simulink model "AD_Stepper"  (Simulink 10.0)
settings: Solver=FixedStepDiscrete  StartTime=0.0  StopTime=inf  FixedStep=Ts  RelTol=1e-3
PostLoadFcn:
  | Ts = 0.01;      % model sample time
  | Tmax = 0.5;   % maximum time per "tick"
libraries: simulink x4, AD_Stepper_motor_lib x2
settings Model: Creator=Admin  LastModifiedBy=bhisma
settings ConfigSet: Description=rtmc9s12target_R2009b
settings DataIOCC: LimitDataPoints=on  SignalLoggingSaveFormat=ModelDataLogs  SaveOutput=off  SaveTime=off  SignalLoggingName=sigsOut
settings OptimizationCC: ExpressionDepthLimit=2147483647  InitFltsAndDblsToZero=on  LifeSpan=1  EfficientTunableParamExpr=on
settings DebuggingCC: SaveWithParameterizedLinksMsg=none  SignalResolutionControl=TryResolveAllWithWarning  MultiTaskDSMMsg=warning  MultiTaskCondExecSysMsg=none  FcnCallInpInsideContextMsg=warning  StateNameClashWarn=warning
settings HardwareCC: ProdBitPerInt=16  ProdBitPerPointer=16  ProdBitPerSizeT=16  ProdBitPerPtrDiffT=16  ProdEndianess=BigEndian  ProdWordSize=16  ProdHWDeviceType=Motorola HC12
settings SFSimCC: MATLABDynamicMemAlloc=off
settings RTWCC: SystemTargetFile=mc9s12.tlc  GenerateMakefile=off  TemplateMakefile=mc9s12.tmf
settings CodeAppCC: CustomSymbolStrType=$N$R$M  InternalIdentifier=Classic
settings STFCustomTargetCC: TargetFcnLib=ansi_tfl_tmw.mat  ModelReferenceCompliant=off  IncludeMdlTerminateFcn=off  ERTCustomFileBanners=on  SupportNonInlinedSFcns=off  RemoveResetFunc=on  MATLABClassNameForMDSCustomization=Simulink.SoftwareTarget.ERTCustomization  CPPClassGenCompliant=on  SystemTargetFile=mc9s12.tlc
settings ERTTargetCC: TargetFcnLib=ansi_tfl_tmw.mat  MultiwordLength=2048  ModelReferenceCompliant=off  ParMdlRefBuildCompliant=off  CompOptLevelCompliant=off  ConcurrentExecutionCompliant=off  IncludeMdlTerminateFcn=off  CombineOutputUpdateFcns=off  SupportContinuousTime=on  ModelStepFunctionPrototypeControlCompliant=off  GRTInterface=on  UseToolchainInfoCompliant=off  ExtModeMexFile=ext_serial_mc9s12_comm  ExtModeMexArgs=1,2,115200  ERTCustomFileTemplate=mc9s12_file_process.tlc  ConvertIfToSwitch=off  SuppressUnreachableDefaultCases=off
settings CustomProperty: DataType=RTWOptions_EnumType_C__Users_fw__SVN_rtmc9s12-target_trunk_rtmc9s12_CW_R2009b_bin_mc9s12_1mc9s12_TargetBoard  Value=Dragon12Plus
settings EnumStrPairs: String=Dragon12
settings ConfigComp: CovExternalEMLEnable=off

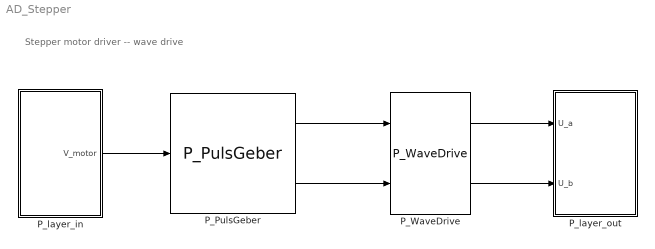
== system AD_Stepper ==
  note: Stepper motor driver -- wave drive
  P_PulsGeber : AD_Stepper_motor_lib/P_PulsGeber  SystemSampleTime=Ts
  P_WaveDrive : AD_Stepper_motor_lib/P_WaveDrive  SystemSampleTime=Ts
  P_layer_in : Subsystem  TreatAsAtomicUnit=on
  P_layer_out : Subsystem  TreatAsAtomicUnit=on  SystemSampleTime=Ts
  wires:
  P_PulsGeber/1 -> P_WaveDrive/1
  P_PulsGeber/2 -> P_WaveDrive/2
  P_layer_in/1(V_motor) -> P_PulsGeber/1
  P_WaveDrive/1 -> P_layer_out/1(U_a)
  P_WaveDrive/2 -> P_layer_out/2(U_b)

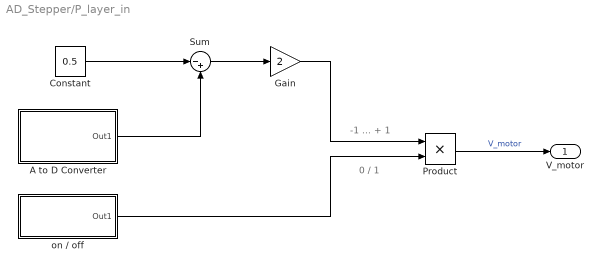
== system AD_Stepper/P_layer_in ==
  note: -1 ... + 1
  note: 0 / 1
  A to D Converter : Subsystem  Tag=mcTarget_adc  mask{bank=0, channels=7, use10bits=10 bits, normalize=max. output:  1, sampletime=Ts}
      mask prompts: bank "ADC bank"; channels "Channels ( 0 - 7 )"; use10bits "ADC resolution"; normalize "Normalization"; sampletime "Sample time"
      mask init:
      | [channelsStr, firstChannel, numChannels] = mbc_adcinput(channels);
      mask Help: web('adc_sfcn_9S12.html');
      mask TypeOptions bank: 0 | 1
      mask TypeOptions use10bits: 10 bits | 8 bits
      mask TypeOptions normalize: raw values | max. output:  1 | max. output:  5
      mask Display: disp(['A to D Converter\n' channelsStr])
  Constant : Constant  Value=0.5
  Gain : Gain  Gain=2
  Product : Product  RndMeth=Zero
  Sum : Sum  Inputs=|-+
  on / off : Subsystem  Tag=mcTarget_digIn  mask{port=Port P, pin=0, sampletime=Ts}
      mask prompts: port "Port (see hardware manuals for valid options)"; pin "Pin (see hardware manuals for valid options)"; sampletime "Sample time"
      mask init:
      | [portstr, pinstr, pins] = mbc_digitalinput(port, pin, sampletime);
      mask Help: web('digIn_sfcn_9S12.html');
      mask TypeOptions port: Port A | Port B | Port H | Port J | Port M | Port P | Port S | Port T
      mask Display: fprintf('%s\nPins: %s', portstr, pinstr)
  V_motor : Outport
  wires:
  Constant/1 -> Sum/1
  A to D Converter/1(Out1) -> Sum/2
  Sum/1 -> Gain/1
  Product/1 -> V_motor/1  "V_motor"
  Gain/1 -> Product/1
  on / off/1(Out1) -> Product/2

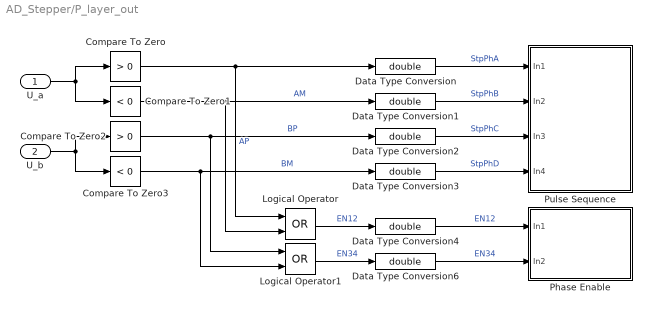
== system AD_Stepper/P_layer_out ==
  U_a : Inport
  U_b : Inport  Port=2
  Compare To Zero : simulink/Logic and Bit Operations/Compare To Zero  SystemSampleTime=-1  relop=>  LogicOutDataTypeMode=boolean  ZeroCross=off
  Compare To Zero1 : simulink/Logic and Bit Operations/Compare To Zero  SystemSampleTime=-1  relop=<  LogicOutDataTypeMode=boolean  ZeroCross=off
  Compare To Zero2 : simulink/Logic and Bit Operations/Compare To Zero  SystemSampleTime=-1  relop=>  LogicOutDataTypeMode=boolean  ZeroCross=off
  Compare To Zero3 : simulink/Logic and Bit Operations/Compare To Zero  SystemSampleTime=-1  relop=<  LogicOutDataTypeMode=boolean  ZeroCross=off
  Data Type Conversion{,1..4,6} (6 alike) : DataTypeConversion  OutDataTypeStr=double
  Logical Operator : Logic  Operator=OR  AllPortsSameDT=off  OutDataTypeStr=boolean
  Logical Operator1 : Logic  Operator=OR  AllPortsSameDT=off  OutDataTypeStr=boolean
  Phase Enable : Subsystem  Tag=mcTarget_digOut  mask{port=Port T, pin=0 1, sampletime=Ts, Von=0.5, Voff=0.5}
      mask prompts: port "Port (see hardware manuals for valid options)"; pin "Pin (see hardware manuals for valid options)"; sampletime "Sample time"; Von "On-threshold (Von)"; Voff "Off-threshold (Voff)"
      mask init:
      | [portstr, pinstr, pins] = mbc_digitaloutput(port, pin, sampletime, Von, Voff);
      mask Help: web('digOut_sfcn_9S12.html');
      mask TypeOptions port: Port A | Port B | Port H | Port J | Port M | Port P | Port S | Port T
      mask Display: fprintf('%s\nPins: %s', portstr, pinstr)
  Pulse Sequence : Subsystem  Tag=mcTarget_digOut  mask{port=Port B, pin=0, 1, 2, 3, sampletime=Ts, Von=0.5, Voff=0.5}
      mask prompts: port "Port (see hardware manuals for valid options)"; pin "Pin (see hardware manuals for valid options)"; sampletime "Sample time"; Von "On-threshold (Von)"; Voff "Off-threshold (Voff)"
      mask init:
      | [portstr, pinstr, pins] = mbc_digitaloutput(port, pin, sampletime, Von, Voff);
      mask Help: web('digOut_sfcn_9S12.html');
      mask TypeOptions port: Port A | Port B | Port H | Port J | Port M | Port P | Port S | Port T
      mask Display: fprintf('%s\nPins: %s', portstr, pinstr)
  wires:
  Data Type Conversion/1 -> Pulse Sequence/1(In1)  "StpPhA"
  Data Type Conversion1/1 -> Pulse Sequence/2(In2)  "StpPhB"
  Data Type Conversion2/1 -> Pulse Sequence/3(In3)  "StpPhC"
  Data Type Conversion3/1 -> Pulse Sequence/4(In4)  "StpPhD"
  Data Type Conversion4/1 -> Phase Enable/1(In1)  "EN12"
  Data Type Conversion6/1 -> Phase Enable/2(In2)  "EN34"
  U_a/1 -> Compare To Zero/1, Compare To Zero1/1
  U_b/1 -> Compare To Zero3/1, Compare To Zero2/1
  Compare To Zero/1 -> Logical Operator/1, Data Type Conversion/1  "AP"
  Compare To Zero1/1 -> Logical Operator/2, Data Type Conversion1/1  "AM"
  Compare To Zero2/1 -> Logical Operator1/1, Data Type Conversion2/1  "BP"
  Compare To Zero3/1 -> Logical Operator1/2, Data Type Conversion3/1  "BM"
  Logical Operator/1 -> Data Type Conversion4/1  "EN12"
  Logical Operator1/1 -> Data Type Conversion6/1  "EN34"

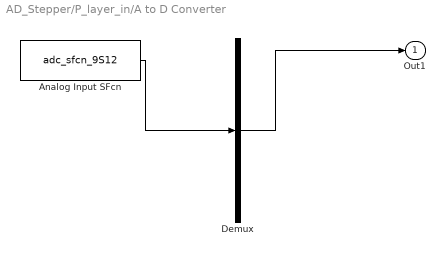
== system AD_Stepper/P_layer_in/A to D Converter ==
  Analog Input SFcn : S-Function  Tag=mcTarget_adc  FunctionName=adc_sfcn_9S12  Parameters=bank-1, firstChannel, numChannels, use10bits-1, normalize, sampletime  SFunctionDeploymentMode=off  EnableBusSupport=off
  Demux : Demux  Outputs=1
  Out1 : Outport
  wires:
  Analog Input SFcn/1 -> Demux/1
  Demux/1 -> Out1/1

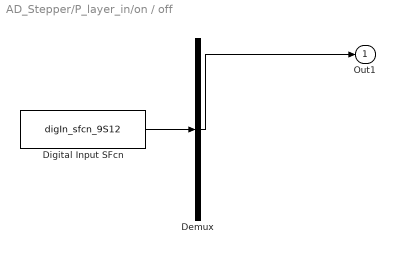
== system AD_Stepper/P_layer_in/on / off ==
  Demux : Demux  Outputs=1
  Digital Input SFcn : S-Function  Tag=mcTarget_digIn  FunctionName=digIn_sfcn_9S12  Parameters=sampletime, port, pins  SFunctionDeploymentMode=off  EnableBusSupport=off
  Out1 : Outport
  wires:
  Demux/1 -> Out1/1
  Digital Input SFcn/1 -> Demux/1

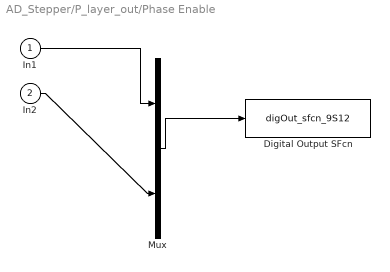
== system AD_Stepper/P_layer_out/Phase Enable ==
  In1 : Inport
  In2 : Inport  Port=2
  Digital Output SFcn : S-Function  Tag=mcTarget_digOut  FunctionName=digOut_sfcn_9S12  Parameters=sampletime, port, pins, Von, Voff  SFunctionDeploymentMode=off  EnableBusSupport=off
  Mux : Mux  Inputs=2
  wires:
  Mux/1 -> Digital Output SFcn/1
  In1/1 -> Mux/1
  In2/1 -> Mux/2

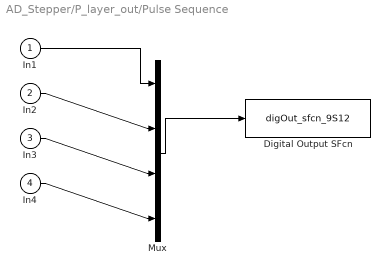
== system AD_Stepper/P_layer_out/Pulse Sequence ==
  In1 : Inport
  In2 : Inport  Port=2
  In3 : Inport  Port=3
  In4 : Inport  Port=4
  Digital Output SFcn : S-Function  Tag=mcTarget_digOut  FunctionName=digOut_sfcn_9S12  Parameters=sampletime, port, pins, Von, Voff  SFunctionDeploymentMode=off  EnableBusSupport=off
  Mux : Mux
  wires:
  Mux/1 -> Digital Output SFcn/1
  In1/1 -> Mux/1
  In2/1 -> Mux/2
  In3/1 -> Mux/3
  In4/1 -> Mux/4
